simulink model "circuitosimetrico"  (Simulink 7.7)
settings: Solver=ode3  StartTime=0  StopTime=0.005  FixedStep=2e-5  RelTol=1e-3
libraries: commfilt2 x1
settings Model: Creator=Cliente  LastModifiedBy=ctu

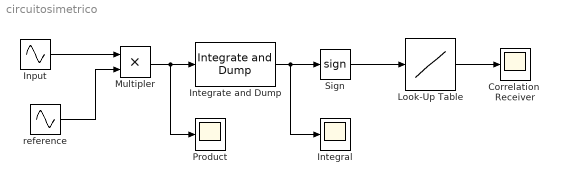
== system circuitosimetrico ==
  Correlation  Receiver : Scope
      settings: SaveName=ScopeData2
  Input : Sin  Frequency=3141.59  SampleTime=20e-6
  Integral : Scope
      settings: YMin=-10  YMax=40
  Integrate and Dump : commfilt2/Integrate and Dump  obssamples=50  offsetsamples=0  nodump=off  roundingMode=Floor  overflowMode=off
  Look-Up Table : Lookup  InputValues=[-1;0;1]  Table=[-1;-1;1]  SaturateOnIntegerOverflow=on
  Multipler : Product  RndMeth=Zero
  Product : Scope
  Sign : Signum
  reference : Sin  Frequency=3141.5926  SampleTime=20e-6
  wires:
  Input/1 -> Multipler/1
  reference/1 -> Multipler/2
  Multipler/1 -> Integrate and Dump/1, Product/1
  Integrate and Dump/1 -> Sign/1, Integral/1
  Sign/1 -> Look-Up Table/1
  Look-Up Table/1 -> Correlation  Receiver/1
